simulink subsystem "filter_sub"  (R2023b)
settings: Solver=VariableStepAuto  StartTime=0.0  StopTime=10.0  RelTol=1e-3
libraries: dspfdesign x3
settings Model: Creator=Edp  LastModifiedBy=giorg

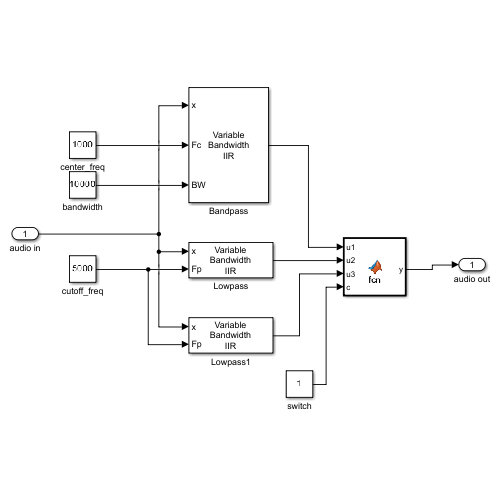
[thumbnail: Simulink's stored preview of the top-level diagram]
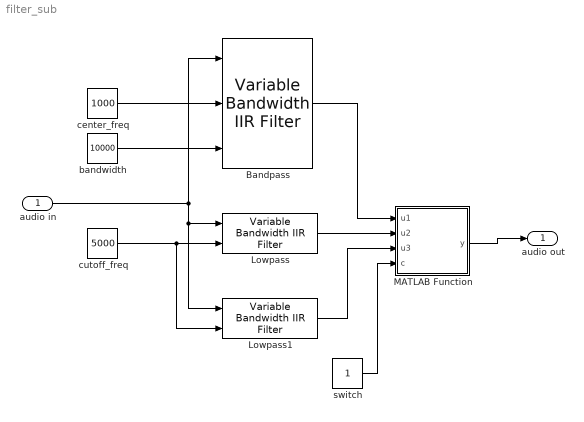
== system filter_sub ==
  audio in : Inport
  Bandpass : dspfdesign/Variable Bandwidth IIR Filter  FilterType=Bandpass  FilterOrder=8  PassbandFrequencyPort=on  PassbandFrequency=512  CenterFrequencyPort=on  CenterFrequency=44100/4  BandwidthPort=on  Bandwidth=7680  PassbandRipple=1  StopbandAttenuation=60  SampleRateMode=Specify on dialog  SampleRate=44100  SimulateUsing=Code generation
  Lowpass : dspfdesign/Variable Bandwidth IIR Filter  FilterType=Lowpass  FilterOrder=8  PassbandFrequencyPort=on  PassbandFrequency=512  CenterFrequencyPort=on  CenterFrequency=44100/4  BandwidthPort=on  Bandwidth=7680  PassbandRipple=1  StopbandAttenuation=60  SampleRateMode=Specify on dialog  SampleRate=44100  SimulateUsing=Code generation
  Lowpass1 : dspfdesign/Variable Bandwidth IIR Filter  FilterType=Highpass  FilterOrder=8  PassbandFrequencyPort=on  PassbandFrequency=512  CenterFrequencyPort=on  CenterFrequency=44100/4  BandwidthPort=on  Bandwidth=7680  PassbandRipple=1  StopbandAttenuation=18  SampleRateMode=Specify on dialog  SampleRate=44100  SimulateUsing=Code generation
  MATLAB Function : MATLAB Function  TreatAsAtomicUnit=on
  bandwidth : Constant  Value=10000
  center_freq : Constant  Value=1000
  cutoff_freq : Constant  Value=5000
  switch : Constant
  audio out : Outport
  wires:
  cutoff_freq/1 -> Lowpass1/2, Lowpass/2
  audio in/1 -> Lowpass1/1, Lowpass/1, Bandpass/1
  center_freq/1 -> Bandpass/2
  Lowpass/1 -> MATLAB Function/2(u2)
  bandwidth/1 -> Bandpass/3
  Bandpass/1 -> MATLAB Function/1(u1)
  MATLAB Function/1(y) -> audio out/1
  switch/1 -> MATLAB Function/4(c)
  Lowpass1/1 -> MATLAB Function/3(u3)

== matlab function filter_sub/MATLAB Function ==
  data: u1 input; y output size=120000; u2 input; u3 input; c input
function y = fcn(u1, u2, u3, c)
y = 0;
if c == 0
    y = u1;
end
if c == 1
    y = u2;
end
if c == 2
    y = u3;
end
